simulink model "VelocityValidation"  (R2022b)
settings: Solver=VariableStepAuto  StartTime=0.0  StopTime=10.0  RelTol=1e-3
StopFcn:
  | inverse_kinematics_func
settings Model: Creator=DELL  LastModifiedBy=DELL

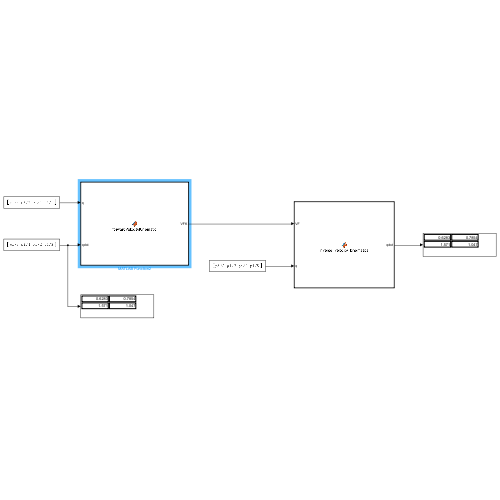
[thumbnail: Simulink's stored preview of the top-level diagram]
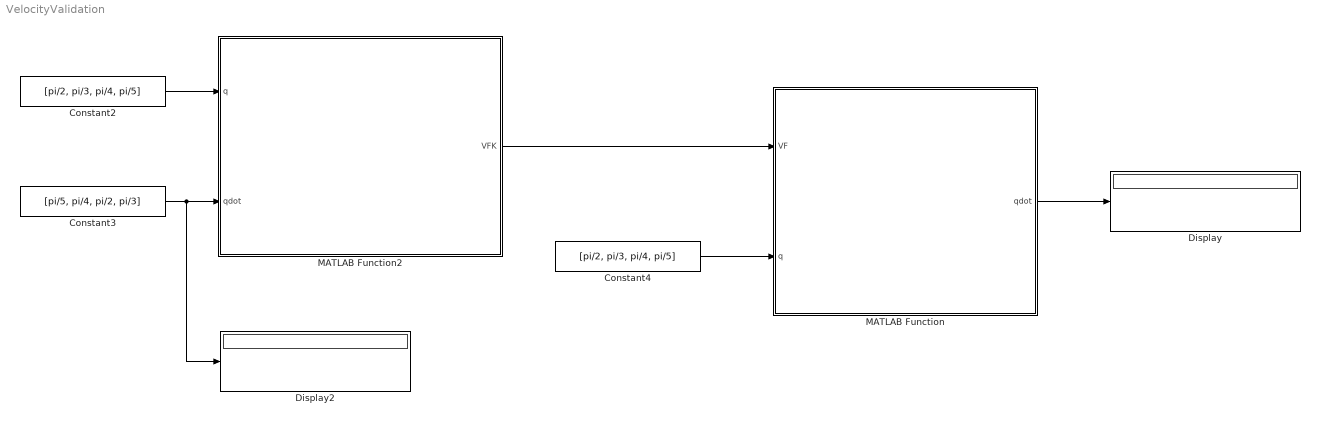
== system VelocityValidation ==
  Constant2 : Constant  Value=[pi/2, pi/3, pi/4, pi/5]
  Constant3 : Constant  Value=[pi/5, pi/4, pi/2, pi/3]
  Constant4 : Constant  Value=[pi/2, pi/3, pi/4, pi/5]
  Display : Display
  Display2 : Display
  MATLAB Function : MATLAB Function  TreatAsAtomicUnit=on
  MATLAB Function2 : MATLAB Function  TreatAsAtomicUnit=on
  wires:
  Constant2/1 -> MATLAB Function2/1(q)
  Constant3/1 -> Display2/1, MATLAB Function2/2(qdot)
  MATLAB Function2/1(VFK) -> MATLAB Function/1(VF)
  Constant4/1 -> MATLAB Function/2(q)
  MATLAB Function/1(qdot) -> Display/1

== matlab function VelocityValidation/MATLAB Function ==
  data: qdot output; VF input; q input
function qdot  = inverse_velocity_kinematics(VF, q)

q1 = q(1);
q2 = q(2);
q3 = q(3);
q4 = q(4);

J =[150*sin(q2)*sin(q1 - pi/2)*sin(q4 - pi/2) - 150*cos(q4 - pi/2)*(cos(q1 - pi/2)*sin(q3 - pi/2) + cos(q2)*cos(q3 - pi/2)*sin(q1 - pi/2)) - 185*sin(q2)*sin(q1 - pi/2),                                                                                                                                                                                                                                                                      -cos(q1 - pi/2)*(150*cos(q2)*sin(q4 - pi/2) - 185*cos(q2) + 150*cos(q3 - pi/2)*cos(q4 - pi/2)*sin(q2)),                                                                                             - cos(q2)*(185*sin(q2)*sin(q1 - pi/2) + 150*cos(q4 - pi/2)*(cos(q1 - pi/2)*sin(q3 - pi/2) + cos(q2)*cos(q3 - pi/2)*sin(q1 - pi/2)) - 150*sin(q2)*sin(q1 - pi/2)*sin(q4 - pi/2)) - sin(q2)*sin(q1 - pi/2)*(150*cos(q2)*sin(q4 - pi/2) - 185*cos(q2) + 150*cos(q3 - pi/2)*cos(q4 - pi/2)*sin(q2)),                                                                                                                - (150*cos(q2)*sin(q4 - pi/2) + 150*cos(q3 - pi/2)*cos(q4 - pi/2)*sin(q2))*(cos(q1 - pi/2)*cos(q3 - pi/2) - cos(q2)*sin(q1 - pi/2)*sin(q3 - pi/2)) - sin(q2)*sin(q3 - pi/2)*(150*cos(q4 - pi/2)*(cos(q1 - pi/2)*sin(q3 - pi/2) + cos(q2)*cos(q3 - pi/2)*sin(q1 - pi/2)) - 150*sin(q2)*sin(q1 - pi/2)*sin(q4 - pi/2));
185*cos(q1 - pi/2)*sin(q2) - 150*cos(q4 - pi/2)*(sin(q1 - pi/2)*sin(q3 - pi/2) - cos(q2)*cos(q1 - pi/2)*cos(q3 - pi/2)) - 150*cos(q1 - pi/2)*sin(q2)*sin(q4 - pi/2),                                                                                                                                                                                                                                                                      -sin(q1 - pi/2)*(150*cos(q2)*sin(q4 - pi/2) - 185*cos(q2) + 150*cos(q3 - pi/2)*cos(q4 - pi/2)*sin(q2)),                                                                                               cos(q1 - pi/2)*sin(q2)*(150*cos(q2)*sin(q4 - pi/2) - 185*cos(q2) + 150*cos(q3 - pi/2)*cos(q4 - pi/2)*sin(q2)) - cos(q2)*(150*cos(q4 - pi/2)*(sin(q1 - pi/2)*sin(q3 - pi/2) - cos(q2)*cos(q1 - pi/2)*cos(q3 - pi/2)) - 185*cos(q1 - pi/2)*sin(q2) + 150*cos(q1 - pi/2)*sin(q2)*sin(q4 - pi/2)),                                                                                                                - (150*cos(q2)*sin(q4 - pi/2) + 150*cos(q3 - pi/2)*cos(q4 - pi/2)*sin(q2))*(cos(q3 - pi/2)*sin(q1 - pi/2) + cos(q2)*cos(q1 - pi/2)*sin(q3 - pi/2)) - sin(q2)*sin(q3 - pi/2)*(150*cos(q4 - pi/2)*(sin(q1 - pi/2)*sin(q3 - pi/2) - cos(q2)*cos(q1 - pi/2)*cos(q3 - pi/2)) + 150*cos(q1 - pi/2)*sin(q2)*sin(q4 - pi/2));
                                                                                                                                                                  0, cos(q1 - pi/2)*(150*cos(q4 - pi/2)*(sin(q1 - pi/2)*sin(q3 - pi/2) - cos(q2)*cos(q1 - pi/2)*cos(q3 - pi/2)) - 185*cos(q1 - pi/2)*sin(q2) + 150*cos(q1 - pi/2)*sin(q2)*sin(q4 - pi/2)) - sin(q1 - pi/2)*(185*sin(q2)*sin(q1 - pi/2) + 150*cos(q4 - pi/2)*(cos(q1 - pi/2)*sin(q3 - pi/2) + cos(q2)*cos(q3 - pi/2)*sin(q1 - pi/2)) - 150*sin(q2)*sin(q1 - pi/2)*sin(q4 - pi/2)), sin(q2)*sin(q1 - pi/2)*(150*cos(q4 - pi/2)*(sin(q1 - pi/2)*sin(q3 - pi/2) - cos(q2)*cos(q1 - pi/2)*cos(q3 - pi/2)) - 185*cos(q1 - pi/2)*sin(q2) + 150*cos(q1 - pi/2)*sin(q2)*sin(q4 - pi/2)) + cos(q1 - pi/2)*sin(q2)*(185*sin(q2)*sin(q1 - pi/2) + 150*cos(q4 - pi/2)*(cos(q1 - pi/2)*sin(q3 - pi/2) + cos(q2)*cos(q3 - pi/2)*sin(q1 - pi/2)) - 150*sin(q2)*sin(q1 - pi/2)*sin(q4 - pi/2)), (150*cos(q4 - pi/2)*(sin(q1 - pi/2)*sin(q3 - pi/2) - cos(q2)*cos(q1 - pi/2)*cos(q3 - pi/2)) + 150*cos(q1 - pi/2)*sin(q2)*sin(q4 - pi/2))*(cos(q1 - pi/2)*cos(q3 - pi/2) - cos(q2)*sin(q1 - pi/2)*sin(q3 - pi/2)) - (150*cos(q4 - pi/2)*(cos(q1 - pi/2)*sin(q3 - pi/2) + cos(q2)*cos(q3 - pi/2)*sin(q1 - pi/2)) - 150*sin(q2)*sin(q1 - pi/2)*sin(q4 - pi/2))*(cos(q3 - pi/2)*sin(q1 - pi/2) + cos(q2)*cos(q1 - pi/2)*sin(q3 - pi/2));
                                                                                                                                                                  0,                                                                                                                                                                                                                                                                                                                                                             -sin(q1 - pi/2),                                                                                                                                                                                                                                                                                                                                                                      cos(q1 - pi/2)*sin(q2),                                                                                                                                                                                                                                                                                                                                                             - cos(q3 - pi/2)*sin(q1 - pi/2) - cos(q2)*cos(q1 - pi/2)*sin(q3 - pi/2);
                                                                                                                                                              0,                                                                                                                                                                                                                                                                                                                                                              cos(q1 - pi/2),                                                                                                                                                                                                                                                                                                                                                                      sin(q2)*sin(q1 - pi/2),                                                                                                                                                                                                                                                                                                                                                               cos(q1 - pi/2)*cos(q3 - pi/2) - cos(q2)*sin(q1 - pi/2)*sin(q3 - pi/2);                                                                                                                                                                  1,                                                                                                                                                                                                                                                                                                                                                                           0,                                                                                                                                                                                                                                                                                                                                                                                     cos(q2),                                                                                                                                                                                                                                                                                                                                                                                                              sin(q2)*sin(q3 - pi/2)];
Jinv = pinv(J);
qdot = Jinv * VF;
end

== matlab function VelocityValidation/MATLAB Function2 ==
  data: VFK output; q input; qdot input
function VFK  = forwardVelocityKinematic(q, qdot)

q1 = q(1);
q2 = q(2);
q3 = q(3);
q4 = q(4);
J =[150*sin(q2)*sin(q1 - pi/2)*sin(q4 - pi/2) - 150*cos(q4 - pi/2)*(cos(q1 - pi/2)*sin(q3 - pi/2) + cos(q2)*cos(q3 - pi/2)*sin(q1 - pi/2)) - 185*sin(q2)*sin(q1 - pi/2),                                                                                                                                                                                                                                                                      -cos(q1 - pi/2)*(150*cos(q2)*sin(q4 - pi/2) - 185*cos(q2) + 150*cos(q3 - pi/2)*cos(q4 - pi/2)*sin(q2)),                                                                                             - cos(q2)*(185*sin(q2)*sin(q1 - pi/2) + 150*cos(q4 - pi/2)*(cos(q1 - pi/2)*sin(q3 - pi/2) + cos(q2)*cos(q3 - pi/2)*sin(q1 - pi/2)) - 150*sin(q2)*sin(q1 - pi/2)*sin(q4 - pi/2)) - sin(q2)*sin(q1 - pi/2)*(150*cos(q2)*sin(q4 - pi/2) - 185*cos(q2) + 150*cos(q3 - pi/2)*cos(q4 - pi/2)*sin(q2)),                                                                                                                - (150*cos(q2)*sin(q4 - pi/2) + 150*cos(q3 - pi/2)*cos(q4 - pi/2)*sin(q2))*(cos(q1 - pi/2)*cos(q3 - pi/2) - cos(q2)*sin(q1 - pi/2)*sin(q3 - pi/2)) - sin(q2)*sin(q3 - pi/2)*(150*cos(q4 - pi/2)*(cos(q1 - pi/2)*sin(q3 - pi/2) + cos(q2)*cos(q3 - pi/2)*sin(q1 - pi/2)) - 150*sin(q2)*sin(q1 - pi/2)*sin(q4 - pi/2));
185*cos(q1 - pi/2)*sin(q2) - 150*cos(q4 - pi/2)*(sin(q1 - pi/2)*sin(q3 - pi/2) - cos(q2)*cos(q1 - pi/2)*cos(q3 - pi/2)) - 150*cos(q1 - pi/2)*sin(q2)*sin(q4 - pi/2),                                                                                                                                                                                                                                                                      -sin(q1 - pi/2)*(150*cos(q2)*sin(q4 - pi/2) - 185*cos(q2) + 150*cos(q3 - pi/2)*cos(q4 - pi/2)*sin(q2)),                                                                                               cos(q1 - pi/2)*sin(q2)*(150*cos(q2)*sin(q4 - pi/2) - 185*cos(q2) + 150*cos(q3 - pi/2)*cos(q4 - pi/2)*sin(q2)) - cos(q2)*(150*cos(q4 - pi/2)*(sin(q1 - pi/2)*sin(q3 - pi/2) - cos(q2)*cos(q1 - pi/2)*cos(q3 - pi/2)) - 185*cos(q1 - pi/2)*sin(q2) + 150*cos(q1 - pi/2)*sin(q2)*sin(q4 - pi/2)),                                                                                                                - (150*cos(q2)*sin(q4 - pi/2) + 150*cos(q3 - pi/2)*cos(q4 - pi/2)*sin(q2))*(cos(q3 - pi/2)*sin(q1 - pi/2) + cos(q2)*cos(q1 - pi/2)*sin(q3 - pi/2)) - sin(q2)*sin(q3 - pi/2)*(150*cos(q4 - pi/2)*(sin(q1 - pi/2)*sin(q3 - pi/2) - cos(q2)*cos(q1 - pi/2)*cos(q3 - pi/2)) + 150*cos(q1 - pi/2)*sin(q2)*sin(q4 - pi/2));
                                                                                                                                                                  0, cos(q1 - pi/2)*(150*cos(q4 - pi/2)*(sin(q1 - pi/2)*sin(q3 - pi/2) - cos(q2)*cos(q1 - pi/2)*cos(q3 - pi/2)) - 185*cos(q1 - pi/2)*sin(q2) + 150*cos(q1 - pi/2)*sin(q2)*sin(q4 - pi/2)) - sin(q1 - pi/2)*(185*sin(q2)*sin(q1 - pi/2) + 150*cos(q4 - pi/2)*(cos(q1 - pi/2)*sin(q3 - pi/2) + cos(q2)*cos(q3 - pi/2)*sin(q1 - pi/2)) - 150*sin(q2)*sin(q1 - pi/2)*sin(q4 - pi/2)), sin(q2)*sin(q1 - pi/2)*(150*cos(q4 - pi/2)*(sin(q1 - pi/2)*sin(q3 - pi/2) - cos(q2)*cos(q1 - pi/2)*cos(q3 - pi/2)) - 185*cos(q1 - pi/2)*sin(q2) + 150*cos(q1 - pi/2)*sin(q2)*sin(q4 - pi/2)) + cos(q1 - pi/2)*sin(q2)*(185*sin(q2)*sin(q1 - pi/2) + 150*cos(q4 - pi/2)*(cos(q1 - pi/2)*sin(q3 - pi/2) + cos(q2)*cos(q3 - pi/2)*sin(q1 - pi/2)) - 150*sin(q2)*sin(q1 - pi/2)*sin(q4 - pi/2)), (150*cos(q4 - pi/2)*(sin(q1 - pi/2)*sin(q3 - pi/2) - cos(q2)*cos(q1 - pi/2)*cos(q3 - pi/2)) + 150*cos(q1 - pi/2)*sin(q2)*sin(q4 - pi/2))*(cos(q1 - pi/2)*cos(q3 - pi/2) - cos(q2)*sin(q1 - pi/2)*sin(q3 - pi/2)) - (150*cos(q4 - pi/2)*(cos(q1 - pi/2)*sin(q3 - pi/2) + cos(q2)*cos(q3 - pi/2)*sin(q1 - pi/2)) - 150*sin(q2)*sin(q1 - pi/2)*sin(q4 - pi/2))*(cos(q3 - pi/2)*sin(q1 - pi/2) + cos(q2)*cos(q1 - pi/2)*sin(q3 - pi/2));
                                                                                                                                                                  0,                                                                                                                                                                                                                                                                                                                                                             -sin(q1 - pi/2),                                                                                                                                                                                                                                                                                                                                                                      cos(q1 - pi/2)*sin(q2),                                                                                                                                                                                                                                                                                                                                                             - cos(q3 - pi/2)*sin(q1 - pi/2) - cos(q2)*cos(q1 - pi/2)*sin(q3 - pi/2);
                                                                                                                                                                  0,                                                                                                                                                                                                                                                                                                                                                              cos(q1 - pi/2),                                                                                                                                                                                                                                                                                                                                                                      sin(q2)*sin(q1 - pi/2),                                                                                                                                                                                                                                                                                                                                                               cos(q1 - pi/2)*cos(q3 - pi/2) - cos(q2)*sin(q1 - pi/2)*sin(q3 - pi/2);                                                                                                                                                                  1,                                                                                                                                                                                                                                                                                                                                                                           0,                                                                                                                                                                                                                                                                                                                                                                                     cos(q2),                                                                                                                                                                                                                                                                                                                                                                                                              sin(q2)*sin(q3 - pi/2)];
 
q1dot = qdot(1);
q2dot = qdot(2);
q3dot = qdot(3); 
q4dot = qdot(4);

VFK = J * [q1dot; q2dot; q3dot; q4dot];
end
